simulink model "fo_sm"  (R2022b)
settings: Solver=VariableStepAuto  StartTime=0.0  StopTime=2  FixedStep=0.01  RelTol=1e-3
libraries: fod x5
settings Model: Creator=张倬境  LastModifiedBy=张倬境
settings DebuggingCC: MaskedZcDiagnostic=none  IgnoredZcDiagnostic=none

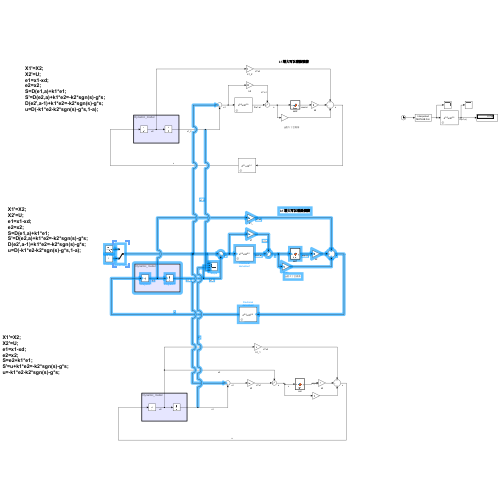
[thumbnail: Simulink's stored preview of the top-level diagram]
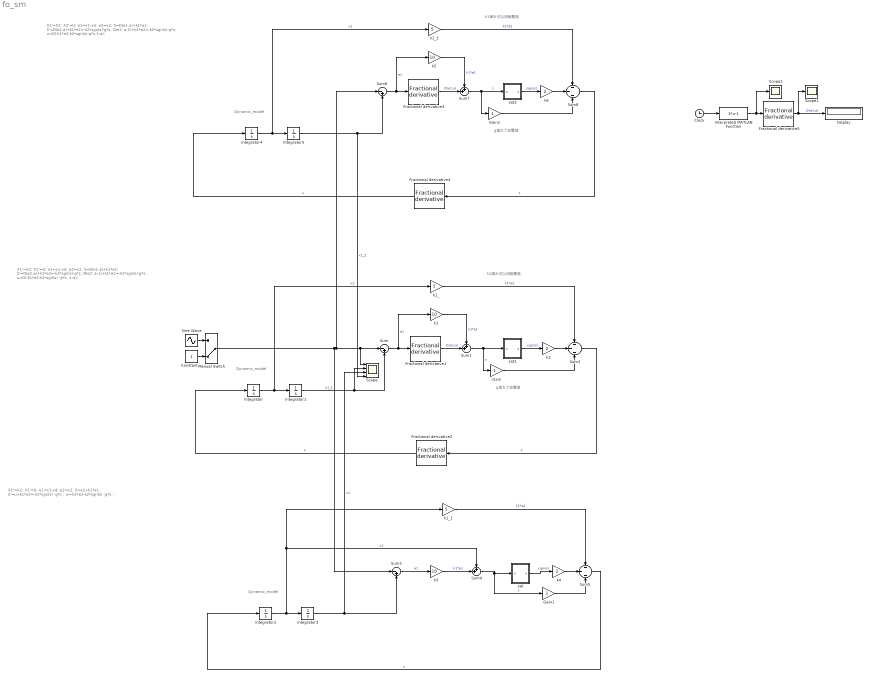
== system fo_sm ==
  note: k1增大可以消除震荡
  note: g值大了会震荡
  note: Dynamic_model
  note: X1'=X2;
      | X2'=U;
      | e1=x1-xd;
      | e2=x2;
      | S=D(e1,a)+k1*e1;
      | S'=D(e2,a)+k1*e2=-k2*sgn(s)-g*s;
      | D(e2',a-1)+k1*e2=-k2*sgn(s)-g*s;
      | u=D(-k1*e2-k2*sgn(s) -g*s ,1-a);
  note: X1'=X2;
      | X2'=U;
      | e1=x1-xd;
      | e2=x2;
      | S=e2+k1*e1;
      | S'=u+k1*e2=-k2*sgn(s) -g*s ;
      | u=-k1*e2-k2*sgn(s) -g*s ;
  note: Dynamic_model
  note: k1增大可以消除震荡
  note: g值大了会震荡
  note: Dynamic_model
  note: X1'=X2;
      | X2'=U;
      | e1=x1-xd;
      | e2=x2;
      | S=D(e1,a)+k1*e1;
      | S'=D(e2,a)+k1*e2=-k2*sgn(s)-g*s;
      | D(e2',a-1)+k1*e2=-k2*sgn(s)-g*s;
      | u=D(-k1*e2-k2*sgn(s)-g*s,1-a);
  Clock : Clock
  Constant : Constant
  Display : Display
  Fractional derivative1 : fod/Fractional derivative  gam=0.5  ww=[0.001; 1000]  n=5  nFod=off
      settings: SourceProductName=FOMCON Toolbox
  Fractional derivative2 : fod/Fractional derivative  gam=0.5  ww=[0.001; 1000]  n=5  nFod=off
      settings: SourceProductName=FOMCON Toolbox
  Fractional derivative3 : fod/Fractional derivative  gam=0.9  ww=[0.001; 1000]  n=5  nFod=off
      settings: SourceProductName=FOMCON Toolbox
  Fractional derivative4 : fod/Fractional derivative  gam=0.1  ww=[0.001; 1000]  n=5  nFod=off
      settings: SourceProductName=FOMCON Toolbox
  Fractional derivative5 : fod/Fractional derivative  gam=0.5  ww=[0.01; 100]  n=10  nFod=off
      settings: SourceProductName=FOMCON Toolbox
  Gain : Gain
  Gain1 : Gain
  Gain2 : Gain
  Integrator{,1..5} (6 alike) : Integrator
  Interpreted MATLAB Function : MATLABFcn  MATLABFcn=2*u-1
  Manual Switch : ManualSwitch  CurrentSetting=0
  Scope : Scope  NumInputPorts=4
  Scope1 : Scope
  Scope2 : Scope
  Sine Wave : Sin  SampleTime=0
  Sum : Sum  Inputs=|-+
  Sum1 : Sum  Inputs=++|
  Sum2 : Sum  Inputs=-|-|-
  Sum3 : Sum  Inputs=|-+
  Sum4 : Sum  Inputs=++|
  Sum5 : Sum  Inputs=-|-|-
  Sum6 : Sum  Inputs=|-+
  Sum7 : Sum  Inputs=++|
  Sum8 : Sum  Inputs=-|-|-
  k1 : Gain  Gain=10
  k1_ : Gain  Gain=5
  k1_1 : Gain  Gain=5
  k1_2 : Gain  Gain=5
  k2 : Gain  Gain=2
  k3 : Gain  Gain=10
  k4 : Gain  Gain=2
  k5 : Gain  Gain=10
  k6 : Gain  Gain=2
  sat : MATLAB Function  TreatAsAtomicUnit=on
  sat1 : MATLAB Function  TreatAsAtomicUnit=on
  sat2 : MATLAB Function  TreatAsAtomicUnit=on
  wires:
  Integrator/1 -> k1_/1, Integrator1/1  "x2"
  Integrator1/1 -> Scope/2, Sum/2  "x1_1"
  Fractional derivative2/1 -> Integrator/1  "u"
  Sum/1 -> k1/1, Fractional derivative1/1  "e1"
  k1/1 -> Sum1/1  "k1*e1"
  Fractional derivative1/1 -> Sum1/2  "D(e1,a)"
  Sum1/1 -> Gain/1, sat1/1(u)  "s"
  k1_/1 -> Sum2/1  "k1*e2"
  k2/1 -> Sum2/2
  Sum2/1 -> Fractional derivative2/1  "s"
  Sum5/1 -> Integrator2/1  "u"
  Sum3/1 -> k3/1  "e1"
  Integrator2/1 -> Sum4/1, k1_1/1, Integrator3/1  "x2"
  Integrator3/1 -> Scope/3, Sum3/2  "x1"
  k3/1 -> Sum4/2  "k1*e1"
  sat1/1(y) -> k2/1  "sign(s)"
  Gain1/1 -> Sum5/3
  sat/1(y) -> k4/1  "sign(s)"
  k4/1 -> Sum5/2
  Sum4/1 -> sat/1(u), Gain1/1  "s"
  k1_1/1 -> Sum5/1  "k1*e2"
  Gain/1 -> Sum2/3
  Constant/1 -> Manual Switch/2
  Sine Wave/1 -> Manual Switch/1
  Manual Switch/1 -> Sum3/1, Sum6/1, Scope/1, Sum/1
  Sum8/1 -> Fractional derivative4/1  "s"
  sat2/1(y) -> k6/1  "sign(s)"
  Sum7/1 -> sat2/1(u), Gain2/1  "s"
  k5/1 -> Sum7/1  "k1*e1"
  Gain2/1 -> Sum8/3
  k6/1 -> Sum8/2
  Fractional derivative3/1 -> Sum7/2  "D(e1,a)"
  Fractional derivative4/1 -> Integrator4/1  "u"
  k1_2/1 -> Sum8/1  "k1*e2"
  Sum6/1 -> k5/1, Fractional derivative3/1  "e1"
  Integrator5/1 -> Sum6/2, Scope/4  "x1_2"
  Integrator4/1 -> k1_2/1, Integrator5/1  "x2"
  Clock/1 -> Interpreted MATLAB Function/1
  Interpreted MATLAB Function/1 -> Scope2/1, Fractional derivative5/1
  Fractional derivative5/1 -> Scope1/1, Display/1  "D(e1,a)"

== matlab function fo_sm/sat ==
  data: u input; y output
function y = fcn(u)
if(abs(u)>0.01)
    y=sign(u);
else   
    y = 100*u;
end
end

== matlab function fo_sm/sat2 ==
  data: u input; y output
function y = fcn(u)
if(abs(u)>0.01)
    y=sign(u);
else   
    y = 100*u;
end
end

== matlab function fo_sm/sat1 ==
  data: u input; y output
function y = fcn(u)
if(abs(u)>0.01)
    y=sign(u);
else   
    y = 100*u;
end
end
